simulink subsystem "Random_generator"  (R2023b)
settings: Solver=VariableStepAuto  StartTime=0.0  StopTime=10.0  RelTol=1e-3
model mask{max_len=20, min_len=15, pitch=0}
values from neighbouring files (symbols this model uses):
  spf_mat = 1024    [inizio.m]    (also in load_preset_audio.m)
undefined symbols (not defined in the file or in its folder): max_grain_size, max_s
libraries: dspsrcs4 x2
settings Model: Creator=Edp  LastModifiedBy=Edp

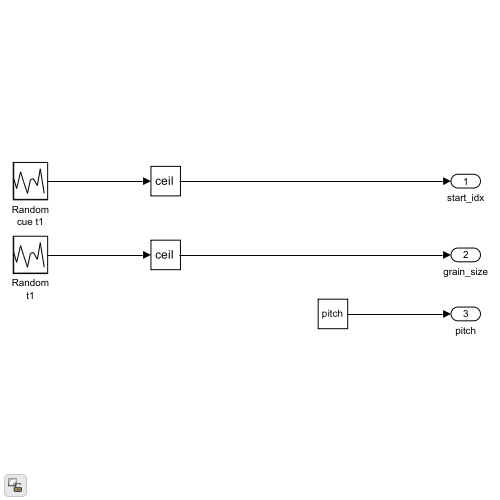
[thumbnail: Simulink's stored preview of the top-level diagram]
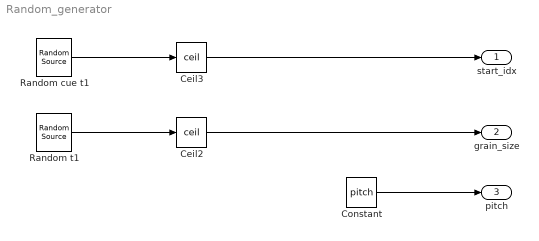
== system Random_generator ==
  Ceil2 : Rounding  Operator=ceil
  Ceil3 : Rounding  Operator=ceil
  Constant : Constant  Value=pitch
  Random cue t1 : dspsrcs4/Random Source  SrcType=Uniform  NormMethod=Ziggurat  CltLength=12  MinVal=1  MaxVal=max_s-max_grain_size*spf_mat  MeanVal=0  VarVal=1  RepMode=Not repeatable  rawSeed=1  IsInherit=off  SampMode=Continuous  SampTime=1  SampFrame=1  DataType=Double  OutComplex=Real  OutputFrames=off
  Random t1 : dspsrcs4/Random Source  SrcType=Uniform  NormMethod=Ziggurat  CltLength=12  MinVal=min_len  MaxVal=max_len  MeanVal=0  VarVal=1  RepMode=Not repeatable  rawSeed=1  IsInherit=off  SampMode=Continuous  SampTime=1  SampFrame=1  DataType=Double  OutComplex=Real  OutputFrames=off
  start_idx : Outport
  grain_size : Outport  Port=2
  pitch : Outport  Port=3
  wires:
  Random t1/1 -> Ceil2/1
  Ceil2/1 -> grain_size/1
  Constant/1 -> pitch/1
  Random cue t1/1 -> Ceil3/1
  Ceil3/1 -> start_idx/1
